simulink model "example1"  (R2013b)
settings: Solver=ode45  StartTime=0.0  StopTime=10.0  RelTol=1e-3
settings Model: Creator=Jin  LastModifiedBy=Jin

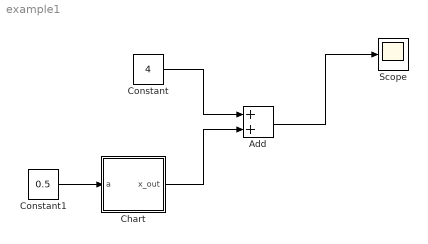
== system example1 ==
  Add : Sum
  Chart : Stateflow chart  TreatAsAtomicUnit=on
  Constant : Constant  Value=4  OutDataTypeStr=double
  Constant1 : Constant  Value=0.5
  Scope : Scope
  wires:
  Constant/1 -> Add/1
  Add/1 -> Scope/1
  Chart/1(x_out) -> Add/2
  Constant1/1 -> Chart/1(a)

== stateflow chart example1/Chart ==
  settings: updateMethod=CONTINUOUS
  state Init
    du:
    x_dot = a;
    x_out = x;
  state Finish
    du:
    x_dot = 0;
    x_out = x;
  (default) -> Init : {x = 1;}
  Init -> Finish : [x >= 7]
  data: x local double; x_out output double; a input double
  data x settings: updateMethod=SF_CONTINUOUS_TIME_DATA
